simulink library "PTOSim_Lib_Updated"  (R2020b)
settings: Solver=ode45  StartTime=0.0  StopTime=10.0  RelTol=1e-3  EnableMultiTasking=on
undefined symbols (not defined in the file or in its folder): DiscIntNeverNeededParam, pAeq, pAupper_limit, pBeq, pBupper_limit, ptosim, table
libraries: simulink x2, $bdroot x1
(part 1 of 2)
settings Model: RequirementInfo="{}  %GIDa_42666abb_d6d9_408c_ae24_f6520282b61c"  Creator=sor  LastModifiedBy=jleonqu
settings DataIOCC: LimitDataPoints=on  SaveFormat=Array  ReturnWorkspaceOutputs=off
settings OptimizationCC: LifeSpan=inf
settings DebuggingCC: SolverPrmCheckMsg=warning  AllowSymbolicDim=off  SFUnexpectedBacktrackingDiag=warning  SFNoUnconditionalDefaultTransitionDiag=warning  SFExecutionAtInitializationDiag=none  ArithmeticOperatorsInVariantConditions=warning
settings HardwareCC: ProdBitPerPointer=32  ProdBitPerSizeT=32  ProdBitPerPtrDiffT=32  ProdLargestAtomicFloat=None  ProdIntDivRoundTo=Undefined  ProdEndianess=Unspecified  ProdWordSize=32  ProdHWDeviceType=32-bit Generic
settings ModelReferenceCC: PropagateSignalLabelsOutOfModel=off
settings SFSimCC: SimUseLocalCustomCode=off  CustomCodeUndefinedFunction=UseInterfaceOnly
settings RTWCC: RTWUseLocalCustomCode=off
settings CodeAppCC: StateflowObjectComments=on
settings GRTTargetCC: TargetLangStandard=C89/C90 (ANSI)
settings ConfigComp: CovMetricSettings=dw  CovSaveCumulativeToWorkspaceVar=on  CovSaveSingleToWorkspaceVar=on  CovExternalEMLEnable=off  CovSFcnEnable=off

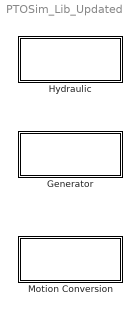
== system PTOSim_Lib_Updated ==
  Generator : Subsystem  RequirementInfo="{}  %GIDa_5439fdb4_7c29_433c_8677_23bf92e18f11"
  Hydraulic : Subsystem  RequirementInfo={} %GIDa_f12a42eb_b9cb_4818_b573_b7dee4183a3b
  Motion Conversion : Subsystem

== system PTOSim_Lib_Updated/Generator ==
  Direct Drive Linear Generator : Subsystem  mask{ptosim=ptosim.pmLinearGenerator(1)}
      mask prompts: ptosim "Machine Name:"
      mask init:
      | if exist ('ptosim','var')
      |     h = [gcb '/To Workspace'];
      |     responseName = ['pmLinearGenerator' num2str(ptosim.number) '_out'];
      |     set_param(h,'VariableName',responseName);
      |     if ischar(ptosim.Rs)==1 ...
      |        || ischar(ptosim.Bfric)==1 ...
      |        || ischar(ptosim.tau_p)==1 ...
      |        || ischar(ptosim.lambda_fd)==1 ...
      |        || ischar(ptosim.Ls)==1 ...
      |        || ischar(ptosim.theta_d_0)==1 ...
      |        || ischar(ptosim.lambda_sq_0)==1 ...
      |        || ischar(ptosim.lambda_sd_0)==1 ...
      |        || ischar(ptosim.Rload) ==1
      |           error('One of the linear generator variables is undefined. For example, ptosim.pmLinearGenerator.variableName')
      |     end       
      | end
      | clear h responseName
  Direct Drive Rotary Generator : Subsystem  RequirementInfo="{}  %GIDa_f3580181_3e4e_42ef_9271_bab532422270"  mask{ptosim=ptosim.pmRotaryGenerator(1)}
      mask prompts: ptosim "Machine Name:"
      mask init:
      | if exist ('ptosim','var')
      |     h = [gcb '/To Workspace'];
      |     responseName = ['pmRotaryGenerator' num2str(ptosim.number) '_out'];
      |     set_param(h,'VariableName',responseName);
      |     if ischar(ptosim.Rs)==1 ...
      |        || ischar(ptosim.Bfric)==1 ...
      |        || ischar(ptosim.tau_p)==1 ...
      |        || ischar(ptosim.lambda_fd)==1 ...
      |        || ischar(ptosim.Ls)==1 ...
      |        || ischar(ptosim.theta_d_0)==1 ...
      |        || ischar(ptosim.lambda_sq_0)==1 ...
      |        || ischar(ptosim.lambda_sd_0)==1 ...
      |        || ischar(ptosim.Rload) ==1 ...
      |        || ischar(ptosim.radius) ==1
      |           error('One of the rotary generator variables is undefined. For example, ptosim.pmRotaryGenerator.variableName')
      |     end       
      | end
      | clear h responseName
  Electric Machine : Subsystem  mask{ptosim=ptosim.ElectricMachine(1), InputFileText=Use PTO-Sim input file to define PTO parameters, Ra=0, La=0, motorConstant=0, ShaftDamping=0, ShaftInertia=0}
      mask prompts: ptosim "Electric Machine Name"; Ra "Armature Resistance [ohm]"; La "Armature Inductance [H]"; motorConstant "Back-emf or Torque constant [V/rpm]"; ShaftDamping "Rotor Damping [N s/m]"; ShaftInertia "Rotor Inertia [kg m^2]"
      settings: PortSchema="{\"entries\":[{\"content\":{\"sides\":[{\"content\":{\"connectorIds\":[\"In1\"]},\"type\":\"ConnectorPlacement.EquallySpacedRectSide\",\"uuid\":\"fc35219d-8831-407a-a01b-8e552e994bd8\"},{\"content\":{\"connectorIds\":[\"Out1\"],\"side\":\"RIGHT\"},\"type\":\"ConnectorPlacement.EquallySpacedRectSide\",\"uuid\":\"8bdf633d-a26b-46f8-9dec-a7b2f777a9d4\"},{\"content\":{\"connectorIds\":[\"In2\"],\"side\":\"TOP\"},\"type\":\"ConnectorPlacement.EquallySpacedRectSide\",\"uuid\":\"317bbc24-ba5c-483d-899e-a231712fee10\"},{\"content\":{\"connectorIds\":[],\"side\":\"HIDDEN\"},\"type\":\"ConnectorPlacement.EquallySpacedRectSide\",\"uuid\":\"59f80c0a-37ef-4cf9-9997-20953bf597e0\"}]},\"type\":\"ConnectorPlacement.EquallySpacedConnector\",\"uuid\":\"aa05d75c-446c-4a7d-9d6c-6346be5c0738\"}],\"packageUris\":[\"http://schema.mathworks.com/mf0/Connector/R2020b\"],\"version\":\"1.0\"}"
      mask DialogControl ParameterGroupVar Prompt: Custom Parameters
      mask DialogControl EMParameters Prompt: Electric Machine Parameters
      mask Display: image('ElectricMotor.png'); % Use "Edit Image" on toolstrip to change.
  Rotary Generator Lookup Table : Subsystem  mask{ptosim=ptosim.rotaryGenerator(1)}
      mask prompts: ptosim "Generator Name"
      mask init:
      | if exist ('ptosim','var')
      |    h = [gcb '/To Workspace'];
      |    responseName = ['rotaryGenerator' num2str(ptosim.number) '_out'];
      |    set_param(h,'VariableName',responseName);
      |    if ischar(ptosim.TgenBase)==1 ...
      |       || ischar(ptosim.omegaBase)==1 ...
      |       || ischar(ptosim.driveEff)==1 ...
      |       || ischar(ptosim.desiredSpeed)==1
      |          error('One of the rotary generator variables is undefined. For example, ptosim.rotaryGenerator.variableName')
      |    end
      | end
      | clear h responseName

== system PTOSim_Lib_Updated/Hydraulic ==
  Accumulator : Subsystem  mask(PTO-Sim Element){ptosim=ptosim.accumulator(1)}
      mask prompts: ptosim "Accumulator Name:"
      mask init:
      | if exist('ptosim','var')
      |     h = [gcb '/To Workspace'];
      |     responseName = ['accumulator' num2str(ptosim.number) '_out'];
      |     set_param(h,'VariableName',responseName);
      |     if ischar(ptosim.VI0)==1 ...
      |             || ischar(ptosim.pIrated)==1 ...
      |             || ischar(ptosim.pIupper_limit)==1 ...
      |             || ischar(ptosim.pIlower_limit)==1 ...
      |             || ischar(ptosim.pIprecharge)==1 ...
      |             || ischar(ptosim.VImax)==1 ...
      |             || ischar(ptosim.VImin)==1 ...
      |             || ischar(ptosim.VIeq)==1 ...
      |             || ischar(ptosim.pIeq)==1 ...
      |             error('One of the accumulator variables is undefined. For example, ptosim.accumulator.variableName')
      |     end
      | end
      | clear h responseName
  Compressible Fluid Piston : Subsystem  mask{ptosim=ptosim.pistonCF(1)}
      mask prompts: ptosim "Piston Name:"
      mask init:
      | if exist ('ptosim','var')
      |     h = [gcb '/To Workspace'];
      |     responseName = ['pistonCF' num2str(ptosim.number) '_out'];
      |     set_param(h,'VariableName',responseName);
      |     
      |     if ischar(ptosim.Ap)==1 ...
      |       || ischar(ptosim.Vo)==1 ...
      |       || ischar(ptosim.Beta_e)==1 ...
      |       || ischar(ptosim.pAi)==1 ...
      |       || ischar(ptosim.pBi)==1 
      |          error('One of the piston variables is undefined. For example, ptosim.pistonCF.variableName')    
      |     end
      | end
      | clear h responseName
  Compressible Fluid Piston Updated : Subsystem  mask{ptosim=ptosim.pistonCF(1), InputFileText=Use PTO-Sim input file to define PTO parameters, Ap_A=0, Ap_B=0, PistonStroke=0, BulkModulus=0, xi_piston=0, pAi=0, pBi=0}
      mask prompts: ptosim "Piston Name"; Ap_A "Piston area A [m]"; Ap_B "Piston area V [m]"; PistonStroke "Piston stroke [m]"; BulkModulus "Fluid Bulk Modulus [Pa]"; xi_piston "Piston initial displacement from A [m]"; pAi "Port A Initial pressure [Pa]"; pBi "Port B Initial pressure [Pa]"
      mask help:
      | PTO-Sim Compressible Fluid Piston
      |
      | This block simualtes a hydraulic cylinder using a compressible fluid model. The block inputs are Response and HydraulicInput. Response is the signal output of the block Rotational PTO Actuation Force. HydraulicInput is a two signal vector with the information of the flow rate for port A and port B of the cylinder. The output of the block is PistonOutput, which is a three signal vector with PressureA, PressureB, and ForcePTO.
      mask init: same as PTOSim_Lib_Updated/Hydraulic/Compressible Fluid Piston
      settings: PortSchema="{\"entries\":[{\"content\":{\"sides\":[{\"content\":{\"connectorIds\":[\"In1\"]},\"type\":\"ConnectorPlacement.EquallySpacedRectSide\",\"uuid\":\"c8df0997-125e-484b-91e1-8ba4eadd9153\"},{\"content\":{\"connectorIds\":[\"Out1\"],\"side\":\"RIGHT\"},\"type\":\"ConnectorPlacement.EquallySpacedRectSide\",\"uuid\":\"941eb644-8b58-45e1-b334-77edb1550c04\"},{\"content\":{\"connectorIds\":[\"In2\"],\"side\":\"TOP\"},\"type\":\"ConnectorPlacement.EquallySpacedRectSide\",\"uuid\":\"a73e5632-eedc-448d-9008-671742bb1d71\"},{\"content\":{\"connectorIds\":[],\"side\":\"HIDDEN\"},\"type\":\"ConnectorPlacement.EquallySpacedRectSide\",\"uuid\":\"aff918e7-82cf-4cd9-bf12-32a09e9272a3\"}]},\"type\":\"ConnectorPlacement.EquallySpacedConnector\",\"uuid\":\"3f3f511d-44ea-4688-8800-5cd126269ecd\"}],\"packageUris\":[\"http://schema.mathworks.com/mf0/Connector/R2020b\"],\"version\":\"1.0\"}"
      mask Help:
      | This block simualtes a hydraulic cylinder using a compressible fluid model. The block inputs are Response and HydraulicInput. Response is the signal output of the block Rotational PTO Actuation Force. HydraulicInput is a two signal vector with the information of the flow rate for port A and port B of the cylinder. The output of the block is PistonOutput, which is a three signal vector with PressureA, PressureB, and ForcePTO.
      | 
      | The outputs are calculated using the model presented in the following link: http://wec-sim.github.io/WEC-Sim/master/user/advanced_features.html#pto-sim
      mask DialogControl ParameterGroupVar Prompt: Custom Parameters
      mask DialogControl PistonProperties Prompt: Piston Properties
      mask DialogControl InitialConditions Prompt: Initial Conditions
      mask Display: image('DoubleActingPiston.png'); % Use "Edit Image" on toolstrip to change.
  Gas-Charged Hydraulic Accumulator : Subsystem  mask{ptosim=ptosim.accumulator(1), InputFileText=Use PTO-Sim input file to define PTO parameters, VI0=0, VIeq=0, pIprecharge=0}
      mask prompts: ptosim "Accumulator Name"; VI0 "Total Volume [m^3]"; VIeq "Initial Volume [m^3]"; pIprecharge "Precharge [Pa]"
      mask DialogControl ParameterGroupVar Prompt: Custom Parameters
      mask DialogControl AccProperties Prompt: Accumulator Properties
      mask Display: image('GasAccumulator.png'); % Use "Edit Image" on toolstrip to change.
  "Hydraulic Motor " : Subsystem  mask{ptosim=ptosim.hydraulicMotor(1)}
      mask prompts: ptosim "Motor Name:"
      mask init:
      | if exist ('ptosim','var')
      |     h = [gcb '/To Workspace'];
      |     responseName = ['hydraulicMotor' num2str(ptosim.number) '_out'];
      |     set_param(h,'VariableName',responseName);
      |     if ischar(ptosim.angVelInit)==1 ...
      |        || ischar(ptosim.J)==1 ...
      |        || ischar(ptosim.fric)==1 ...
      |           error('One of the motor variables is undefined. For example, ptosim.hydraulicMotor.variableName')
      |     end       
      | end
      | clear h responseName
  Noncompressible Fluid Piston : Subsystem  mask{ptosim=ptosim.pistonNCF(1)}
      mask prompts: ptosim "Piston Name:"
      mask init:
      | if exist ('ptosim','var')
      |     h = [gcb '/To Workspace'];
      |     responseName = ['pistonNCF' num2str(ptosim.number) '_out'];
      |     set_param(h,'VariableName',responseName);
      |     if ischar(ptosim.topA)==1 ...
      |       || ischar(ptosim.botA)==1
      |          error('One of the piston variables is undefined. For example, ptosim.pistonNCF.variableName')
      |     end
      | end
      | clear h responseName
  Rectifying Check Valve : Subsystem  mask{ptosim=ptosim.checkValve(1)}
      mask prompts: ptosim "Valve Name:"
      mask init:
      | if exist ('ptosim','var')
      |     h = [gcb '/To Workspace'];
      |     responseName = ['checkValve' num2str(ptosim.number) '_out'];
      |     set_param(h,'VariableName',responseName);
      |     
      |     if ischar(ptosim.Cd)==1 ...
      |        || ischar(ptosim.Amax)==1 ...
      |        || ischar(ptosim.Amin)==1 ...
      |        || ischar(ptosim.pMax)==1 ...
      |        || ischar(ptosim.pMin)==1 ...
      |        || ischar(ptosim.rho)==1 ...
      |        || ischar(ptosim.k1)==1 ...
      |        || ischar(ptosim.k2)==1 
      |           error('One of valve variables is undefined. For exmaple, ptosim.checkValve.variableName')
      |     end
      | end
      | clear h responseName
  Rectifying Valve : Subsystem  mask{ptosim=ptosim.valve(1)}
      mask prompts: ptosim "Valve Name:"
      mask init:
      | if exist ('ptosim','var')
      |     h = [gcb '/To Workspace'];
      |     responseName = ['valve' num2str(ptosim.number) '_out'];
      |     set_param(h,'VariableName',responseName);
      | end
      | clear h responseName

== system PTOSim_Lib_Updated/Motion Conversion ==
  Rotary to Linear Adjustable Rod : Subsystem  mask{ptosim=ptosim.motionMechanism(1)}
      mask prompts: ptosim "Telescope Name:"
      mask init:
      | if exist('ptosim','var')
      |     h = [gcb '/To Workspace'];
      |     responseName = ['motionMechanism' num2str(ptosim.number) '_out'];
      |     set_param(h,'VariableName',responseName);
      |     if ischar(ptosim.crank)==1 ...
      |             || ischar(ptosim.rodInit)==1 ...
      |             || ischar(ptosim.offset)==1 ...
      |             error('One of the rotary to linear adjustable rod variables is undefined. For example, ptosim.motionMechanism.variableName')
      |     end
      | end
      | clear h responseName
  Rotary to Linear Crank : Subsystem  mask{ptosim=ptosim.motionMechanism(1)}
      mask prompts: ptosim "Crank Name:"
      mask init:
      | if exist('ptosim','var')
      |     h = [gcb '/To Workspace'];
      |     responseName = ['motionMechanism' num2str(ptosim.number) '_out'];
      |     set_param(h,'VariableName',responseName);
      |     if ischar(ptosim.crank)==1 ...
      |             || ischar(ptosim.rodLength)==1 ...
      |             || ischar(ptosim.offset)==1 ...
      |             error('One of the rotary to linear crank variables is undefined. For example, ptosim.motionMechanism.variableName')
      |     end
      | end
      | clear h responseName

== system PTOSim_Lib_Updated/Generator/Direct Drive Linear Generator ==
  note: In this model d-axis aligned with rotor magnets
      | in other words lambda_fq = 0
  note: Ls = 3/2*Lsinglephase
  vel : Inport
  ABC2DQ1 : Subsystem
  ABC2DQ2 : Subsystem
  Bus Creator : BusCreator  Inputs=11
  Demux : Demux  Outputs=3
  Demux1 : Demux  Outputs=3
  Gain4 : Gain  Gain=-1
  Gain5 : Gain  Gain=2*pi/(2*ptosim.tau_p)
  Integrator2 : Integrator  InitialCondition=ptosim.theta_d_0
  Load : Subsystem
  Losses : Subsystem
  Product1 : Product
  Subsystem : Subsystem
  Sum : Sum
  Terminator3 : Terminator
  To Workspace : ToWorkspace  VariableName=pmLinearGenerator1_out  SaveFormat=Structure With Time  SampleTime=-1
      settings: Decimation=round(simu.dtOut/simu.dt,0)
  force : Outport
  wires:
  ABC2DQ2/1(DQ) -> Subsystem/1(vsdq)  "vsdq"
  ABC2DQ1/1(abc) -> Demux/1, Load/1(Iabc)  "Iabc"
  Gain5/1 -> Subsystem/2(wd), Integrator2/1  "wsyn"
  Integrator2/1 -> ABC2DQ2/1(theta_d), ABC2DQ1/1(theta_d)
  Product1/1 -> Gain4/1
  Gain4/1 -> Bus Creator/1, Terminator3/1  "absPower"
  Subsystem/1(Fem) -> Sum/2
  Subsystem/2(isdq) -> ABC2DQ1/2(dq)
  Losses/1(friceForce) -> Bus Creator/3, Sum/1  "fricForce"
  Sum/1 -> Bus Creator/2, Product1/2, force/1  "force"
  Load/1(Vabc) -> Demux1/1, ABC2DQ2/2(ABC)  "Vabc"
  vel/1 -> Bus Creator/10, Losses/1(vel), Product1/1, Gain5/1  "vel"
  Bus Creator/1 -> To Workspace/1
  Demux/1 -> Bus Creator/4  "Ia"
  Demux/2 -> Bus Creator/5  "Ib"
  Demux/3 -> Bus Creator/6  "Ic"
  Demux1/1 -> Bus Creator/7  "Va"
  Demux1/2 -> Bus Creator/8  "Vb"
  Demux1/3 -> Bus Creator/9  "Vc"
  Load/2(elecPower) -> Bus Creator/11  "elecPower"

== system PTOSim_Lib_Updated/Generator/Direct Drive Rotary Generator ==
  note: In this model d-axis aligned with rotor magnets
      | in other words lambda_fq = 0
  note: Ls = 3/2*Lsinglephase
  vel : Inport
  ABC2DQ1 : Subsystem
  ABC2DQ2 : Subsystem
  Bus Creator : BusCreator  Inputs=11
  Demux : Demux  Outputs=3
  Demux1 : Demux  Outputs=3
  Gain4 : Gain  Gain=-1
  Gain5 : Gain  Gain=2*pi*ptosim.radius/(2*ptosim.tau_p)
  Integrator2 : Integrator  InitialCondition=ptosim.theta_d_0
  Load : Subsystem
  Losses : Subsystem
  Product1 : Product
  Subsystem : Subsystem
  Sum : Sum
  Terminator3 : Terminator
  To Workspace : ToWorkspace  VariableName=pmRotaryGenerator1_out  SaveFormat=Structure With Time  SampleTime=-1
      settings: Decimation=round(simu.dtOut/simu.dt,0)
  torque : Outport
  wires:
  ABC2DQ2/1(DQ) -> Subsystem/1(vsdq)  "vsdq"
  ABC2DQ1/1(abc) -> Demux/1, Load/1(Iabc)  "Iabc"
  Gain5/1 -> Integrator2/1, Subsystem/2(wd)  "wsyn"
  Integrator2/1 -> ABC2DQ2/1(theta_d), ABC2DQ1/1(theta_d)
  Product1/1 -> Gain4/1
  Gain4/1 -> Bus Creator/1, Terminator3/1  "absPower"
  Subsystem/1(Tem) -> Sum/2
  Subsystem/2(isdq) -> ABC2DQ1/2(dq)
  Losses/1(fricTorque) -> Bus Creator/3, Sum/1  "fricTorque"
  Sum/1 -> Bus Creator/2, Product1/2, torque/1  "torque"
  Load/1(Vabc) -> Demux1/1, ABC2DQ2/2(ABC)  "Vabc"
  vel/1 -> Losses/1(vel), Product1/1, Gain5/1, Bus Creator/10  "vel"
  Bus Creator/1 -> To Workspace/1
  Demux/1 -> Bus Creator/4  "Ia"
  Demux/2 -> Bus Creator/5  "Ib"
  Demux/3 -> Bus Creator/6  "Ic"
  Demux1/1 -> Bus Creator/7  "Va"
  Demux1/2 -> Bus Creator/8  "Vb"
  Demux1/3 -> Bus Creator/9  "Vc"
  Load/2(elecPower) -> Bus Creator/11  "elecPower"

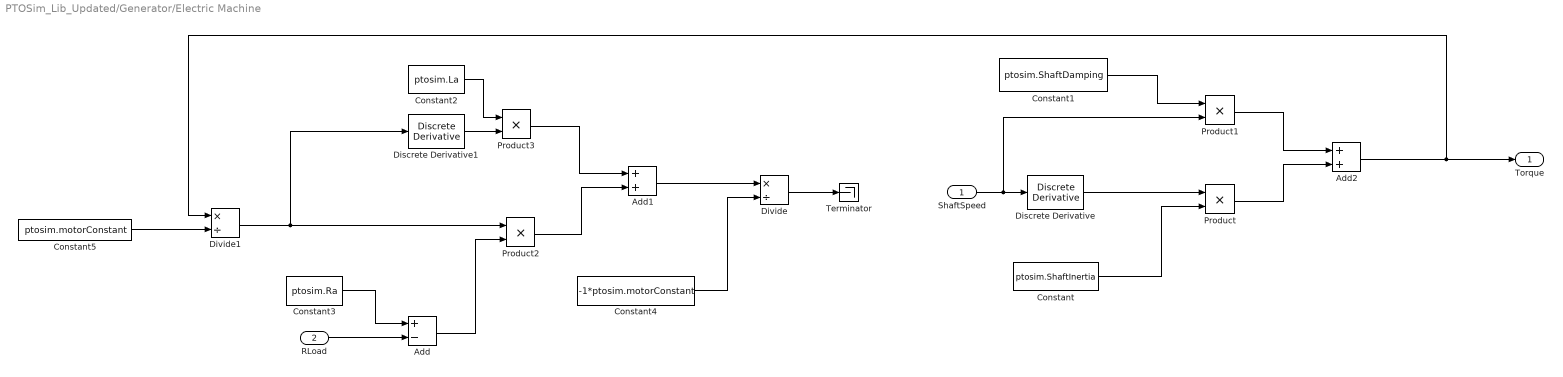
== system PTOSim_Lib_Updated/Generator/Electric Machine ==
  ShaftSpeed : Inport
  RLoad : Inport  Port=2
  Add : Sum  Inputs=+-
  Add1 : Sum
  Add2 : Sum
  Constant : Constant  Value=ptosim.ShaftInertia
  Constant1 : Constant  Value=ptosim.ShaftDamping
  Constant2 : Constant  Value=ptosim.La
  Constant3 : Constant  Value=ptosim.Ra
  Constant4 : Constant  Value=-1*ptosim.motorConstant
  Constant5 : Constant  Value=ptosim.motorConstant
  Discrete Derivative : simulink/Discrete/Discrete Derivative  gainval=1.0  ICPrevScaledInput=0.0  OutMin=[]  OutMax=[]  OutDataType=fixdt(1, 16)  OutScaling=2^-10  DoSatur=off
  Discrete Derivative1 : simulink/Quick Insert/Discrete/Discrete Derivative  gainval=1.0  ICPrevScaledInput=0.0  OutMin=[]  OutMax=[]  OutDataType=fixdt(1, 16)  OutScaling=2^-10  DoSatur=off
      settings: SourceProductBaseCode=SL
  Divide : Product  Inputs=*/
  Divide1 : Product  Inputs=*/
  Product{,1..3} (4 alike) : Product
  Terminator : Terminator
  Torque : Outport
  wires:
  Discrete Derivative/1 -> Product/1
  Constant/1 -> Product/2
  Constant1/1 -> Product1/1
  Divide1/1 -> Discrete Derivative1/1, Product2/1
  RLoad/1 -> Add/2
  Constant3/1 -> Add/1
  Add/1 -> Product2/2
  Discrete Derivative1/1 -> Product3/2
  Constant2/1 -> Product3/1
  Product3/1 -> Add1/1
  Product2/1 -> Add1/2
  Add1/1 -> Divide/1
  Constant4/1 -> Divide/2
  Product1/1 -> Add2/1
  Product/1 -> Add2/2
  Add2/1 -> Divide1/1, Torque/1
  ShaftSpeed/1 -> Product1/2, Discrete Derivative/1
  Constant5/1 -> Divide1/2
  Divide/1 -> Terminator/1

== system PTOSim_Lib_Updated/Generator/Rotary Generator Lookup Table ==
  delPress : Inport
  motorVol : Inport  Port=2
  angVel : Inport  Port=3
  Base Motor Torque : Gain  Gain=-1/ptosim.TgenBase
  Base Motor Torque1 : Gain  Gain=1/ptosim.omegaBase
  Base Motor Torque2 : Gain  Gain=ptosim.driveEff
  Base Motor Torque3 : Gain  Gain=1/100
  Base Motor Torque4 : Gain  Gain=1.05
  Bus Creator : BusCreator  Inputs=2
  Constant47 : Constant  Value=ptosim.desiredSpeed
  Divide1 : Product  Inputs=*/
  PM p.u. Efficiency Lookup Table : Lookup_n-D  BreakpointsForDimension1=table.Tpu(:,1)  BreakpointsForDimension2=table.omegapu(1,:)  Table=table.eff  InterpMethod=Flat  InputSameDT=on
      settings: InputPortMap=u0,u1
  Product{,1..3} (4 alike) : Product  RndMeth=Zero
  To Workspace : ToWorkspace  VariableName=rotaryGenerator1_out  SaveFormat=Structure With Time  SampleTime=-1
      settings: Decimation=round(simu.dtOut/simu.dt,0)
  genTorque : Outport
  wires:
  angVel/1 -> Product2/2, Product/2, Base Motor Torque1/1
  Product2/1 -> Product/1, Base Motor Torque/1, genTorque/1
  Bus Creator/1 -> To Workspace/1
  Base Motor Torque/1 -> PM p.u. Efficiency Lookup Table/1  "torquePU"
  Base Motor Torque1/1 -> PM p.u. Efficiency Lookup Table/2  "omegaPU"
  PM p.u. Efficiency Lookup Table/1 -> Base Motor Torque3/1
  Base Motor Torque3/1 -> Product1/2  "genEff"
  Product/1 -> Product1/1, Bus Creator/2  "genPower"
  Product1/1 -> Base Motor Torque2/1
  Base Motor Torque2/1 -> Bus Creator/1  "elecPower"
  Divide1/1 -> Product2/1
  delPress/1 -> Product3/1
  motorVol/1 -> Product3/2
  Product3/1 -> Divide1/1
  Constant47/1 -> Base Motor Torque4/1
  Base Motor Torque4/1 -> Divide1/2

== system PTOSim_Lib_Updated/Hydraulic/Accumulator ==
  volFlowM : Inport
  volFlowAccum : Inport  Port=2
  Bus Creator : BusCreator  Inputs=2
  Constant : Constant
  Constant3 : Constant  Value=ptosim.pIprecharge
  Constant4 : Constant  Value=ptosim.VI0
  Divide : Product  Inputs=*/
  Divide1 : Product  Inputs=*/
  Exponent : Constant  Value=1.4
  Integrator4 : Integrator  InitialCondition=ptosim.VIeq
  Math Function : Math  Operator=pow  SignedPower=on  SaturateOnIntegerOverflow=on
  Sum : Sum  Inputs=-+
  Sum2 : Sum
  To Workspace : ToWorkspace  VariableName=accum_out  SaveFormat=Structure With Time  SampleTime=-1
      settings: Decimation=round(simu.dtOut/simu.dt,0)
  pressure : Outport
  wires:
  Sum2/1 -> Integrator4/1
  Integrator4/1 -> Bus Creator/2, Divide/1  "volume"
  Constant4/1 -> Divide/2
  Constant/1 -> Sum/2
  Divide/1 -> Sum/1
  Exponent/1 -> Math Function/2
  Sum/1 -> Math Function/1
  Math Function/1 -> Divide1/2
  Constant3/1 -> Divide1/1
  Divide1/1 -> pressure/1, Bus Creator/1  "pressure"
  volFlowAccum/1 -> Sum2/2
  volFlowM/1 -> Sum2/1
  Bus Creator/1 -> To Workspace/1

== system PTOSim_Lib_Updated/Hydraulic/Compressible Fluid Piston ==
  pos : Inport
  vel : Inport  Port=2
  volFlowTop : Inport  Port=3
  volFlowBottom : Inport  Port=4
  Bus Creator : BusCreator  Inputs=4
  Gain1 : Gain  Gain=-1
  Gain6 : Gain  Gain=ptosim.Ap
  Gain7 : Gain  Gain=ptosim.Ap
  Pressure Bottom : Subsystem
  Pressure Top : Subsystem
  Product : Product
  Sum4 : Sum  Inputs=-+
  To Workspace : ToWorkspace  VariableName=pistonCF1_out  SaveFormat=Structure With Time  SampleTime=-1
      settings: Decimation=round(simu.dtOut/simu.dt,0)
  force : Outport
  topPressure : Outport  Port=2
  bottomPressure : Outport  Port=3
  wires:
  Pressure Top/1(topPressure) -> Sum4/1, topPressure/1
  Pressure Bottom/1(bottomPressure) -> bottomPressure/1, Sum4/2
  Gain7/1 -> Pressure Bottom/3(volFLowP), Pressure Top/3(volFlowP)
  pos/1 -> Bus Creator/3, Pressure Bottom/1(pos), Pressure Top/1(pos)  "pos"
  vel/1 -> Bus Creator/4, Product/2, Gain7/1  "vel"
  Sum4/1 -> Gain6/1
  Gain6/1 -> Bus Creator/2, force/1, Product/1  "force"
  volFlowBottom/1 -> Pressure Bottom/2(volFlowBottom)
  volFlowTop/1 -> Pressure Top/2(volFlowTop)
  Bus Creator/1 -> To Workspace/1
  Gain1/1 -> Bus Creator/1  "absPower"
  Product/1 -> Gain1/1

== system PTOSim_Lib_Updated/Hydraulic/Compressible Fluid Piston Updated ==
  HydraulicInput : Inport
  Response : Inport  Port=2
  Add : Sum  Inputs=-+
  Bus Creator : BusCreator  Inputs=3
  Bus Selector : BusSelector  OutputSignals=position,velocity
  Bus Selector1 : BusSelector  OutputSignals=QA,QB
  Constant : Constant  Value=ptosim.Ap_B
  Constant1 : Constant  Value=ptosim.Ap_A
  Discrete-Time Integrator : DiscreteIntegrator  InitialCondition=ptosim.pAi  SampleTime=-1  ICPrevOutput=DiscIntNeverNeededParam  ICPrevScaledInput=DiscIntNeverNeededParam
  Discrete-Time Integrator1 : DiscreteIntegrator  InitialCondition=ptosim.pBi  SampleTime=-1  ICPrevOutput=DiscIntNeverNeededParam  ICPrevScaledInput=DiscIntNeverNeededParam
  Product1 : Product
  Product2 : Product
  Selector : Selector  InputPortWidth=6  IndexOptions=Index vector (dialog)  Indices=3  OutputSizes=1
  Selector1 : Selector  InputPortWidth=6  IndexOptions=Index vector (dialog)  Indices=3  OutputSizes=1
  Subsystem : Subsystem  AncestorBlock=PTOSim_Lib_Updated/Hydraulic/Compressible Fluid Piston Updated/Subsystem
  dPa_dt : Subsystem  AncestorBlock=PTOSim_Lib_Updated/Hydraulic/Compressible Fluid Piston Updated/dPa_dt
  PistonOutput : Outport
  wires:
  Bus Selector/1 -> Selector/1  "<position>"
  Product1/1 -> Add/2
  HydraulicInput/1 -> Bus Selector1/1
  Subsystem/1(dPB_dt) -> Discrete-Time Integrator1/1
  dPa_dt/1(dPA_dt) -> Discrete-Time Integrator/1
  Product2/1 -> Add/1
  Selector/1 -> Subsystem/1(Pos), dPa_dt/1(Pos)
  Discrete-Time Integrator/1 -> Bus Creator/1, Product2/1  "PressureA"
  Response/1 -> Bus Selector/1
  Selector1/1 -> Subsystem/2(Vel), dPa_dt/2(Vel)
  Discrete-Time Integrator1/1 -> Bus Creator/3, Product1/2  "ForcePTO"
  Bus Selector/2 -> Selector1/1  "<velocity>"
  Constant/1 -> Product1/1
  Constant1/1 -> Product2/2
  Add/1 -> Bus Creator/2  "PressureB"
  Bus Creator/1 -> PistonOutput/1
  Bus Selector1/2 -> Subsystem/3(QB)  "<QB>"
  Bus Selector1/1 -> dPa_dt/3(QA)  "<QA>"

== system PTOSim_Lib_Updated/Hydraulic/Gas-Charged Hydraulic Accumulator ==
  FlowRate : Inport
  Add : Sum  Inputs=+-
  Constant : Constant  Value=ptosim.VI0
  Constant1 : Constant
  Constant2 : Constant  Value=1.4
  Constant3 : Constant  Value=ptosim.pIprecharge
  Discrete-Time Integrator : DiscreteIntegrator  InitialCondition=ptosim.VIeq  SampleTime=-1  ICPrevOutput=DiscIntNeverNeededParam  ICPrevScaledInput=DiscIntNeverNeededParam
  Divide : Product  Inputs=*/
  Divide1 : Product  Inputs=*/
  Math Function : Math  Operator=pow  SaturateOnIntegerOverflow=on
  Pressure : Outport
  wires:
  FlowRate/1 -> Discrete-Time Integrator/1
  Discrete-Time Integrator/1 -> Divide/1
  Constant/1 -> Divide/2
  Divide/1 -> Add/2
  Constant1/1 -> Add/1
  Add/1 -> Math Function/1
  Constant2/1 -> Math Function/2
  Math Function/1 -> Divide1/2
  Constant3/1 -> Divide1/1
  Divide1/1 -> Pressure/1

== system PTOSim_Lib_Updated/Hydraulic/Hydraulic Motor  ==
  highPressure : Inport
  lowPressure : Inport  Port=2
  genTorque : Inport  Port=3
  Bus Creator : BusCreator  Inputs=2
  Constant47 : Constant  Value=ptosim.J
  Divide1 : Product  Inputs=*/
  Gain1 : Gain  Gain=ptosim.fric
  Gain4 : Gain  Gain=-1
  Integrator1 : Integrator  InitialCondition=ptosim.angVelInit
  Interpreted MATLAB Function : MATLABFcn  MATLABFcn=variableMotorVolume
  Product : Product
  Product1 : Product
  Sum1 : Sum  Inputs=+--
  Sum2 : Sum  Inputs=+-
  To Workspace : ToWorkspace  VariableName=hydraulicMotor1_out  SaveFormat=Structure With Time  SampleTime=-1
      settings: Decimation=round(simu.dtOut/simu.dt,0)
  delPress : Outport
  motorVol : Outport  Port=2
  angVel : Outport  Port=3
  volFlowMHigh : Outport  Port=4
  volFlowMLow : Outport  Port=5
  wires:
  Interpreted MATLAB Function/1 -> motorVol/1, Product/2, Product1/2
  Sum2/1 -> delPress/1, Product/1, Interpreted MATLAB Function/1
  Gain1/1 -> Sum1/3
  genTorque/1 -> Sum1/2, Gain1/1
  Bus Creator/1 -> To Workspace/1
  Gain4/1 -> volFlowMHigh/1
  lowPressure/1 -> Sum2/2
  highPressure/1 -> Sum2/1
  Integrator1/1 -> angVel/1, Product1/1, Bus Creator/1  "angVel"
  Divide1/1 -> Integrator1/1
  Constant47/1 -> Divide1/2
  Sum1/1 -> Divide1/1
  Product/1 -> Sum1/1
  Product1/1 -> volFlowMLow/1, Gain4/1, Bus Creator/2  "volFlowM"

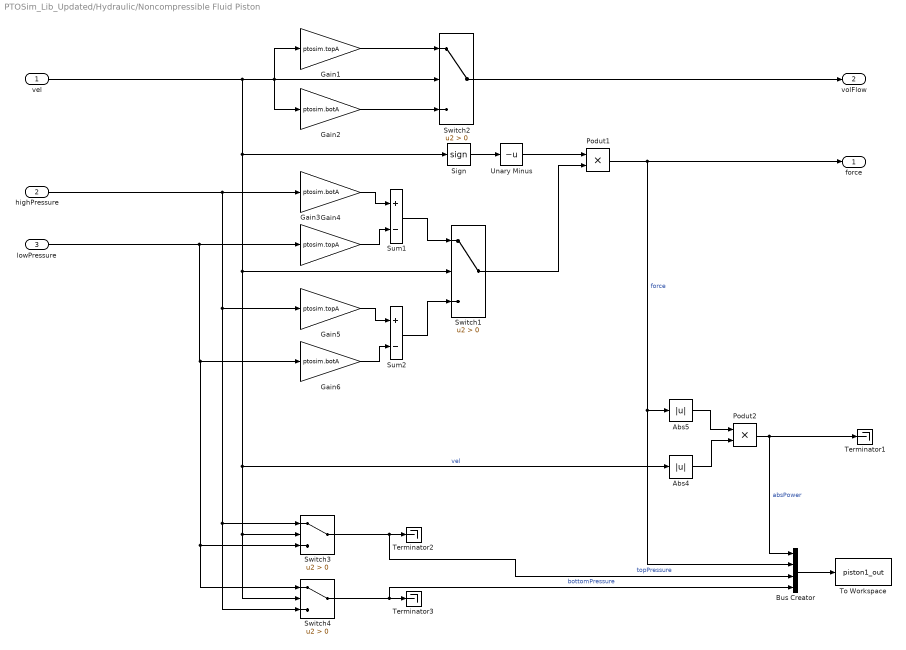
== system PTOSim_Lib_Updated/Hydraulic/Noncompressible Fluid Piston ==
  vel : Inport
  highPressure : Inport  Port=2
  lowPressure : Inport  Port=3
  Abs4 : Abs
  Abs5 : Abs
  Bus Creator : BusCreator  Inputs=4
  Gain1 : Gain  Gain=ptosim.topA
  Gain2 : Gain  Gain=ptosim.botA
  Gain3 : Gain  Gain=ptosim.topA
  Gain4 : Gain  Gain=ptosim.botA
  Gain5 : Gain  Gain=ptosim.topA
  Gain6 : Gain  Gain=ptosim.botA
  Podut1 : Product  RndMeth=Zero
  Podut2 : Product  RndMeth=Zero
  Sign : Signum
  Sum1 : Sum  Inputs=+-
  Sum2 : Sum  Inputs=+-
  Switch{1..4} (4 alike) : Switch  Criteria=u2 > Threshold
  Terminator1 : Terminator
  Terminator2 : Terminator
  Terminator3 : Terminator
  To Workspace : ToWorkspace  VariableName=piston1_out  SaveFormat=Structure With Time  SampleTime=-1
      settings: Decimation=round(simu.dtOut/simu.dt,0)
  Unary Minus : UnaryMinus
  force : Outport
  volFlow : Outport  Port=2
  wires:
  vel/1 -> Switch1/2, Switch4/2, Switch3/2, Abs4/1, Sign/1, Gain2/1, Switch2/2, Gain1/1  "vel"
  Podut2/1 -> Bus Creator/1, Terminator1/1  "absPower"
  Abs5/1 -> Podut2/1
  Abs4/1 -> Podut2/2
  Gain1/1 -> Switch2/1
  Gain2/1 -> Switch2/3
  Sum1/1 -> Switch1/1
  Podut1/1 -> force/1, Bus Creator/2, Abs5/1  "force"
  Gain4/1 -> Sum1/1
  Gain3/1 -> Sum1/2
  highPressure/1 -> Gain5/1, Switch3/1, Switch4/3, Gain4/1
  lowPressure/1 -> Switch4/1, Switch3/3, Gain6/1, Gain3/1
  Gain5/1 -> Sum2/1
  Gain6/1 -> Sum2/2
  Sum2/1 -> Switch1/3
  Sign/1 -> Unary Minus/1
  Unary Minus/1 -> Podut1/1
  Switch1/1 -> Podut1/2
  Switch3/1 -> Bus Creator/3, Terminator2/1  "topPressure"
  Switch4/1 -> Bus Creator/4, Terminator3/1  "bottomPressure"
  Switch2/1 -> volFlow/1
  Bus Creator/1 -> To Workspace/1

== system PTOSim_Lib_Updated/Hydraulic/Rectifying Check Valve ==
  topPressure : Inport
  bottomPressure : Inport  Port=2
  highPressure : Inport  Port=3
  lowPressure : Inport  Port=4
  Bus Creator : BusCreator  Inputs=4
  Subsystem : Subsystem
  Subsystem1 : Subsystem
  Subsystem2 : Subsystem
  Subsystem3 : Subsystem
  Sum1 : Sum  Inputs=-+
  Sum2 : Sum
  Sum3 : Sum  Inputs=--
  Sum4 : Sum  Inputs=-+
  To Workspace : ToWorkspace  VariableName=valve1_out  SaveFormat=Structure With Time  SampleTime=-1
      settings: Decimation=round(simu.dtOut/simu.dt,0)
  volFlowTop : Outport
  volFlowBottom : Outport  Port=2
  volFlowHigh : Outport  Port=3
  volFlowLow : Outport  Port=4
  wires:
  topPressure/1 -> Subsystem3/2(topPressure), Subsystem/1(topPressure)
  bottomPressure/1 -> Subsystem2/2(bottomPressure), Subsystem1/1(bottomPressure)
  highPressure/1 -> Subsystem1/2(highPressure), Subsystem/2(highPressure)
  lowPressure/1 -> Subsystem2/1(lowPressure), Subsystem3/1(lowPressure)
  Subsystem3/1(volFlow4) -> Bus Creator/4, Sum4/2, Sum3/2  "volFlow4"
  Subsystem2/1(volFlow3) -> Bus Creator/3, Sum3/1, Sum1/2  "volFlow3"
  Subsystem1/1(volFlow2) -> Bus Creator/2, Sum2/2, Sum1/1  "volFlow2"
  Subsystem/1(volFlow1) -> Bus Creator/1, Sum2/1, Sum4/1  "volFlow1"
  Sum4/1 -> volFlowTop/1
  Sum1/1 -> volFlowBottom/1
  Sum2/1 -> volFlowHigh/1
  Sum3/1 -> volFlowLow/1
  Bus Creator/1 -> To Workspace/1

== system PTOSim_Lib_Updated/Hydraulic/Rectifying Valve ==
  volFlow : Inport
  Abs1 : Abs
  To Workspace : ToWorkspace  VariableName=valve1_out  SaveFormat=Structure With Time  SampleTime=-1
      settings: Decimation=round(simu.dtOut/simu.dt,0)
  electric generator control1 : Gain  Gain=-1
  volFlowHigh : Outport
  volFlowLow : Outport  Port=2
  wires:
  Abs1/1 -> To Workspace/1, volFlowHigh/1, electric generator control1/1  "volFlow"
  electric generator control1/1 -> volFlowLow/1
  volFlow/1 -> Abs1/1

== system PTOSim_Lib_Updated/Motion Conversion/Rotary to Linear Adjustable Rod ==
  angPos : Inport
  angVel : Inport  Port=2
  force : Inport  Port=3
  Add : Sum
  Angle Calculation for PTO : Subsystem
  Angular to Linear Position : Subsystem
  Angular to Linear Velocity : Subsystem
  Bus Creator : BusCreator  Inputs=3
  Constant1 : Constant  Value=ptosim.crank
  Constant2 : Constant  Value=ptosim.crank
  Gain : Gain  Gain=-1
  Product : Product  Inputs=4
  Product1 : Product  Inputs=4
  To Workspace : ToWorkspace  VariableName=motionmech1_out  SaveFormat=Structure With Time  SampleTime=-1
      settings: Decimation=round(simu.dtOut/simu.dt,0)
  Trigonometric Function : Trigonometry
  Trigonometric Function1 : Trigonometry  Operator=cos
  linearPos : Outport
  linearVel : Outport  Port=2
  torque : Outport  Port=3
  wires:
  Angular to Linear Position/1(linearPos) -> linearPos/1
  angVel/1 -> Bus Creator/3, Angular to Linear Velocity/2(angVel)  "angVelocity"
  Angular to Linear Velocity/1(linearVel) -> linearVel/1
  Add/1 -> Bus Creator/1, torque/1  "ptoTorque"
  Bus Creator/1 -> To Workspace/1
  angPos/1 -> Angular to Linear Velocity/1(angPos), Trigonometric Function1/1, Trigonometric Function/1, Angle Calculation for PTO/1(angPos), Bus Creator/2, Angular to Linear Position/1(angPos)  "angPosition"
  Product1/1 -> Add/1
  Gain/1 -> Add/2
  Angle Calculation for PTO/2(Sin_gamma) -> Product/1
  Trigonometric Function1/1 -> Product1/3
  Angle Calculation for PTO/1(Cos_gamma) -> Product1/1
  force/1 -> Product1/4, Product/4
  Constant2/1 -> Product1/2
  Trigonometric Function/1 -> Product/3
  Constant1/1 -> Product/2
  Product/1 -> Gain/1

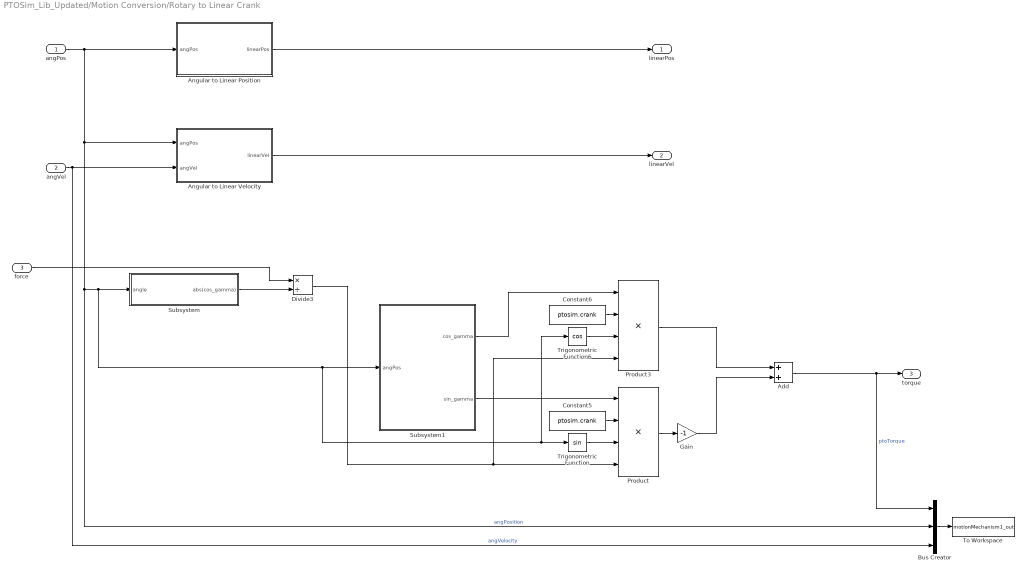
== system PTOSim_Lib_Updated/Motion Conversion/Rotary to Linear Crank ==
  angPos : Inport
  angVel : Inport  Port=2
  force : Inport  Port=3
  Add : Sum
  Angular to Linear Position : Subsystem
  Angular to Linear Velocity : Subsystem
  Bus Creator : BusCreator  Inputs=3
  Constant5 : Constant  Value=ptosim.crank
  Constant6 : Constant  Value=ptosim.crank
  Divide3 : Product  Inputs=*/
  Gain : Gain  Gain=-1
  Product : Product  Inputs=4
  Product3 : Product  Inputs=4
  Subsystem : Subsystem
  Subsystem1 : Subsystem  AncestorBlock=PTOSim_Lib/Motion Conversion/Rotary to Linear Adjustable Rod/Subsystem
  To Workspace : ToWorkspace  VariableName=motionMechanism1_out  SaveFormat=Structure With Time  SampleTime=-1
      settings: Decimation=round(simu.dtOut/simu.dt,0)
  Trigonometric Function : Trigonometry
  Trigonometric Function6 : Trigonometry  Operator=cos
  linearPos : Outport
  linearVel : Outport  Port=2
  torque : Outport  Port=3
  wires:
  Angular to Linear Position/1(linearPos) -> linearPos/1
  angVel/1 -> Bus Creator/3, Angular to Linear Velocity/2(angVel)  "angVelocity"
  Angular to Linear Velocity/1(linearVel) -> linearVel/1
  Add/1 -> Bus Creator/1, torque/1  "ptoTorque"
  Bus Creator/1 -> To Workspace/1
  Subsystem/1(abs(cos_gamma)) -> Divide3/2
  force/1 -> Divide3/1
  Trigonometric Function6/1 -> Product3/3
  Subsystem1/1(cos_gamma) -> Product3/1
  Constant6/1 -> Product3/2
  Divide3/1 -> Product/4, Product3/4
  Gain/1 -> Add/2
  Product3/1 -> Add/1
  Subsystem1/2(sin_gamma) -> Product/1
  angPos/1 -> Angular to Linear Velocity/1(angPos), Subsystem1/1(angPos), Trigonometric Function/1, Trigonometric Function6/1, Subsystem/1(angle), Bus Creator/2, Angular to Linear Position/1(angPos)  "angPosition"
  Trigonometric Function/1 -> Product/3
  Constant5/1 -> Product/2
  Product/1 -> Gain/1

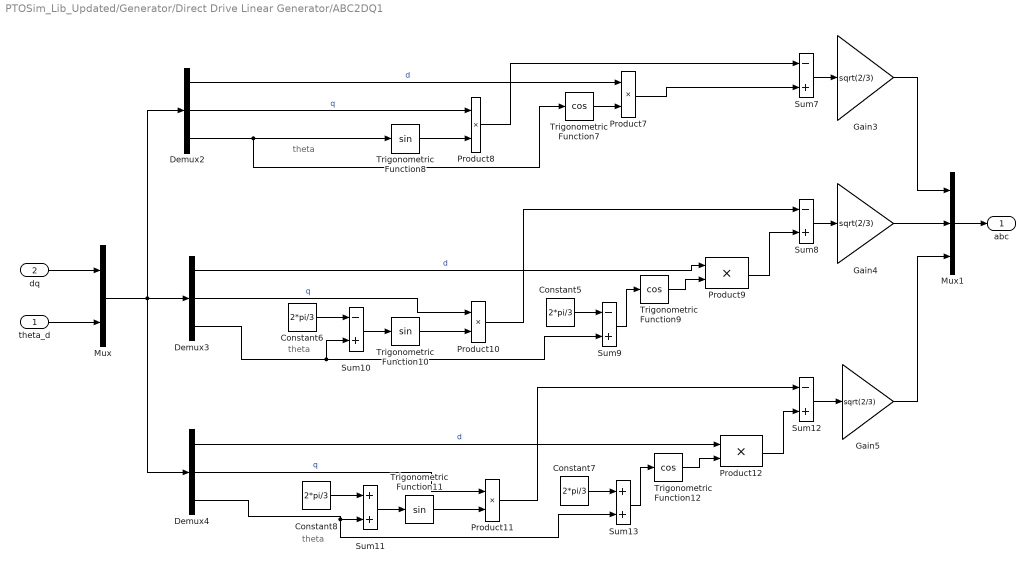
== system PTOSim_Lib_Updated/Generator/Direct Drive Linear Generator/ABC2DQ1 ==
  note: theta
  note: theta
  note: theta
  theta_d : Inport
  dq : Inport  Port=2
  Constant{5..8} (4 alike) : Constant  Value=2*pi/3
  Demux2 : Demux  Outputs=3
      settings: DisplayOption=none
  Demux3 : Demux  Outputs=3
      settings: DisplayOption=none
  Demux4 : Demux  Outputs=3
      settings: DisplayOption=none
  Gain3 : Gain  Gain=sqrt(2/3)  SaturateOnIntegerOverflow=on  OutDataTypeStr=Inherit: Same as input  ParamDataTypeStr=Inherit: Same as input
  Gain4 : Gain  Gain=sqrt(2/3)  SaturateOnIntegerOverflow=on  OutDataTypeStr=Inherit: Same as input  ParamDataTypeStr=Inherit: Same as input
  Gain5 : Gain  Gain=sqrt(2/3)  SaturateOnIntegerOverflow=on  OutDataTypeStr=Inherit: Same as input  ParamDataTypeStr=Inherit: Same as input
  Mux : Mux  Inputs=2
  Mux1 : Mux  Inputs=3
  Product{7..12} (6 alike) : Product  InputSameDT=on  SaturateOnIntegerOverflow=on  OutDataTypeStr=Inherit: Same as first input
  Sum{7..10,12} (5 alike) : Sum  Inputs=-+  InputSameDT=on  SaturateOnIntegerOverflow=on  OutDataTypeStr=Inherit: Same as first input
  Sum11 : Sum  InputSameDT=on  SaturateOnIntegerOverflow=on  OutDataTypeStr=Inherit: Same as first input
  Sum13 : Sum  InputSameDT=on  SaturateOnIntegerOverflow=on  OutDataTypeStr=Inherit: Same as first input
  Trigonometric Function10 : Trigonometry
  Trigonometric Function11 : Trigonometry
  Trigonometric Function12 : Trigonometry  Operator=cos
  Trigonometric Function7 : Trigonometry  Operator=cos
  Trigonometric Function8 : Trigonometry
  Trigonometric Function9 : Trigonometry  Operator=cos
  abc : Outport
  wires:
  Mux1/1 -> abc/1
  dq/1 -> Mux/1
  theta_d/1 -> Mux/2
  Mux/1 -> Demux4/1, Demux2/1, Demux3/1
  Trigonometric Function7/1 -> Product7/2
  Demux2/1 -> Product7/1  "d"
  Product7/1 -> Sum7/2
  Product8/1 -> Sum7/1
  Demux2/3 -> Trigonometric Function8/1, Trigonometric Function7/1
  Demux2/2 -> Product8/1  "q"
  Trigonometric Function9/1 -> Product9/2
  Demux3/1 -> Product9/1  "d"
  Product9/1 -> Sum8/2
  Product10/1 -> Sum8/1
  Demux3/3 -> Sum10/2, Sum9/2
  Trigonometric Function10/1 -> Product10/2
  Demux3/2 -> Product10/1  "q"
  Sum9/1 -> Trigonometric Function9/1
  Constant5/1 -> Sum9/1
  Sum10/1 -> Trigonometric Function10/1
  Constant6/1 -> Sum10/1
  Trigonometric Function12/1 -> Product12/2
  Demux4/1 -> Product12/1  "d"
  Product12/1 -> Sum12/2
  Product11/1 -> Sum12/1
  Demux4/3 -> Sum13/2, Sum11/2
  Trigonometric Function11/1 -> Product11/2
  Demux4/2 -> Product11/1  "q"
  Sum13/1 -> Trigonometric Function12/1
  Constant7/1 -> Sum13/1
  Sum11/1 -> Trigonometric Function11/1
  Constant8/1 -> Sum11/1
  Sum7/1 -> Gain3/1
  Sum8/1 -> Gain4/1
  Sum12/1 -> Gain5/1
  Gain3/1 -> Mux1/1
  Gain4/1 -> Mux1/2
  Gain5/1 -> Mux1/3
  Trigonometric Function8/1 -> Product8/2

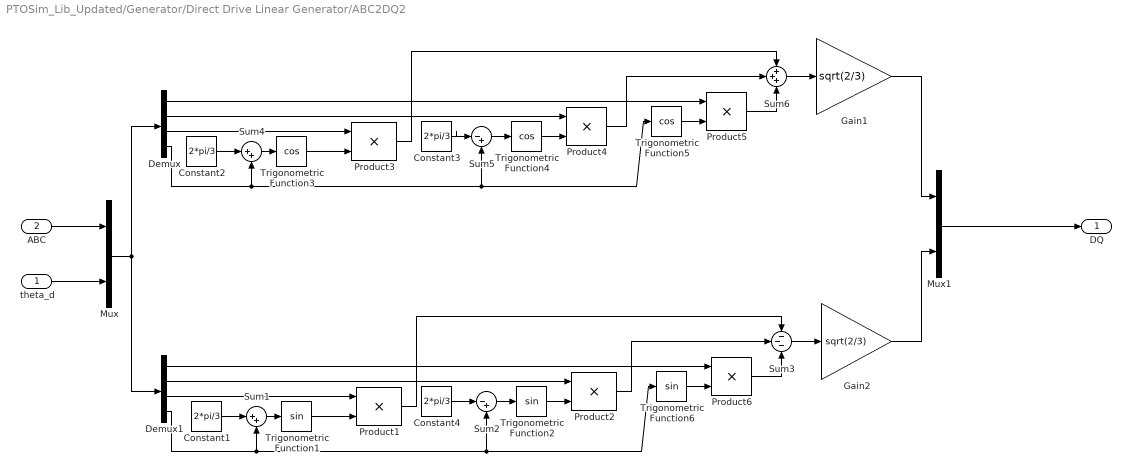
== system PTOSim_Lib_Updated/Generator/Direct Drive Linear Generator/ABC2DQ2 ==
  theta_d : Inport
  ABC : Inport  Port=2
  Constant{1..4} (4 alike) : Constant  Value=2*pi/3
  Demux : Demux
      settings: DisplayOption=none
  Demux1 : Demux
      settings: DisplayOption=none
  Gain1 : Gain  Gain=sqrt(2/3)  SaturateOnIntegerOverflow=on  OutDataTypeStr=Inherit: Same as input  ParamDataTypeStr=Inherit: Same as input
  Gain2 : Gain  Gain=sqrt(2/3)  SaturateOnIntegerOverflow=on  OutDataTypeStr=Inherit: Same as input  ParamDataTypeStr=Inherit: Same as input
  Mux : Mux  Inputs=2
  Mux1 : Mux  Inputs=2
  Product{1..6} (6 alike) : Product  InputSameDT=on  SaturateOnIntegerOverflow=on  OutDataTypeStr=Inherit: Same as first input
  Sum1 : Sum  Inputs=|++  InputSameDT=on  SaturateOnIntegerOverflow=on  OutDataTypeStr=Inherit: Same as first input
  Sum2 : Sum  Inputs=|-+  InputSameDT=on  SaturateOnIntegerOverflow=on  OutDataTypeStr=Inherit: Same as first input
  Sum3 : Sum  Inputs=---  InputSameDT=on  SaturateOnIntegerOverflow=on  OutDataTypeStr=Inherit: Same as first input
  Sum4 : Sum  Inputs=|++  InputSameDT=on  SaturateOnIntegerOverflow=on  OutDataTypeStr=Inherit: Same as first input
  Sum5 : Sum  Inputs=|-+  InputSameDT=on  SaturateOnIntegerOverflow=on  OutDataTypeStr=Inherit: Same as first input
  Sum6 : Sum  Inputs=+++  InputSameDT=on  SaturateOnIntegerOverflow=on  OutDataTypeStr=Inherit: Same as first input
  Trigonometric Function1 : Trigonometry
  Trigonometric Function2 : Trigonometry
  Trigonometric Function3 : Trigonometry  Operator=cos
  Trigonometric Function4 : Trigonometry  Operator=cos
  Trigonometric Function5 : Trigonometry  Operator=cos
  Trigonometric Function6 : Trigonometry
  DQ : Outport
  wires:
  Mux1/1 -> DQ/1
  Product5/1 -> Sum6/3
  Constant2/1 -> Sum4/1
  Sum5/1 -> Trigonometric Function4/1
  Trigonometric Function4/1 -> Product4/2
  Trigonometric Function5/1 -> Product5/2
  Constant3/1 -> Sum5/1
  Sum6/1 -> Gain1/1
  Product3/1 -> Sum6/1
  Product4/1 -> Sum6/2
  Trigonometric Function3/1 -> Product3/2
  Gain1/1 -> Mux1/1
  ABC/1 -> Mux/1
  theta_d/1 -> Mux/2
  Demux/1 -> Product5/1
  Demux/2 -> Product4/1
  Demux/3 -> Product3/1
  Demux/4 -> Sum5/2, Trigonometric Function5/1, Sum4/2
  Mux/1 -> Demux/1, Demux1/1
  Sum4/1 -> Trigonometric Function3/1
  Product6/1 -> Sum3/3
  Constant1/1 -> Sum1/1
  Sum2/1 -> Trigonometric Function2/1
  Trigonometric Function2/1 -> Product2/2
  Trigonometric Function6/1 -> Product6/2
  Constant4/1 -> Sum2/1
  Sum3/1 -> Gain2/1
  Product1/1 -> Sum3/1
  Product2/1 -> Sum3/2
  Trigonometric Function1/1 -> Product1/2
  Gain2/1 -> Mux1/2
  Demux1/1 -> Product6/1
  Demux1/2 -> Product2/1
  Demux1/3 -> Product1/1
  Demux1/4 -> Sum1/2, Trigonometric Function6/1, Sum2/2
  Sum1/1 -> Trigonometric Function1/1

== system PTOSim_Lib_Updated/Generator/Direct Drive Linear Generator/Load ==
  Iabc : Inport
  Gain : Gain  Gain=-1
  Gain1 : Gain  Gain=ptosim.Rload
  Product : Product
  Sum of Elements : Sum  Inputs=+
  Vabc : Outport
  elecPower : Outport  Port=2
  wires:
  Gain/1 -> elecPower/1  "elecPower"
  Gain1/1 -> Product/1, Vabc/1
  Product/1 -> Sum of Elements/1
  Iabc/1 -> Gain1/1, Product/2
  Sum of Elements/1 -> Gain/1

== system PTOSim_Lib_Updated/Generator/Direct Drive Linear Generator/Losses ==
  vel : Inport
  Gain : Gain  Gain=ptosim.Bfric
  friceForce : Outport
  wires:
  vel/1 -> Gain/1
  Gain/1 -> friceForce/1

== system PTOSim_Lib_Updated/Generator/Direct Drive Linear Generator/Subsystem ==
  vsdq : Inport
  wd : Inport  Port=2
  Add : Sum  Inputs=+-+
  Add1 : Sum  Inputs=--+
  Demux2 : Demux  Outputs=2
      settings: DisplayOption=none
  Fcn : Fcn  Expr=( u(1) - ptosim.lambda_fd ) / ptosim.Ls
  Gain : Gain  Gain=1/ptosim.Ls
  Gain1 : Gain  Gain=pi/ptosim.tau_p*ptosim.lambda_fd
  Gain2 : Gain  Gain=ptosim.Rs
  Gain3 : Gain  Gain=ptosim.Rs
  Integrator : Integrator  InitialCondition=ptosim.lambda_sd_0
  Integrator1 : Integrator  InitialCondition=ptosim.lambda_sq_0
  Mux : Mux  Inputs=2
  Product : Product  RndMeth=Zero
  Product1 : Product  RndMeth=Zero
  Fem : Outport
  isdq : Outport  Port=2
  wires:
  Add/1 -> Integrator/1  "d_dt_lambda_sd"
  Integrator/1 -> Product1/2, Fcn/1  "lambda_sd"
  Fcn/1 -> Gain3/1, Mux/1  "isd"
  Product/1 -> Add/1
  Add1/1 -> Integrator1/1  "d_dt_lambda_sq"
  Integrator1/1 -> Gain/1, Product/2  "lambda_sq"
  wd/1 -> Product1/1, Product/1
  Gain/1 -> Gain2/1, Mux/2, Gain1/1  "isq"
  Product1/1 -> Add1/1
  Demux2/1 -> Add/3  "vsd"
  Demux2/2 -> Add1/3  "vsq"
  vsdq/1 -> Demux2/1  "vsdq"
  Gain3/1 -> Add/2  "isd_Rs"
  Gain2/1 -> Add1/2
  Mux/1 -> isdq/1  "isdq"
  Gain1/1 -> Fem/1

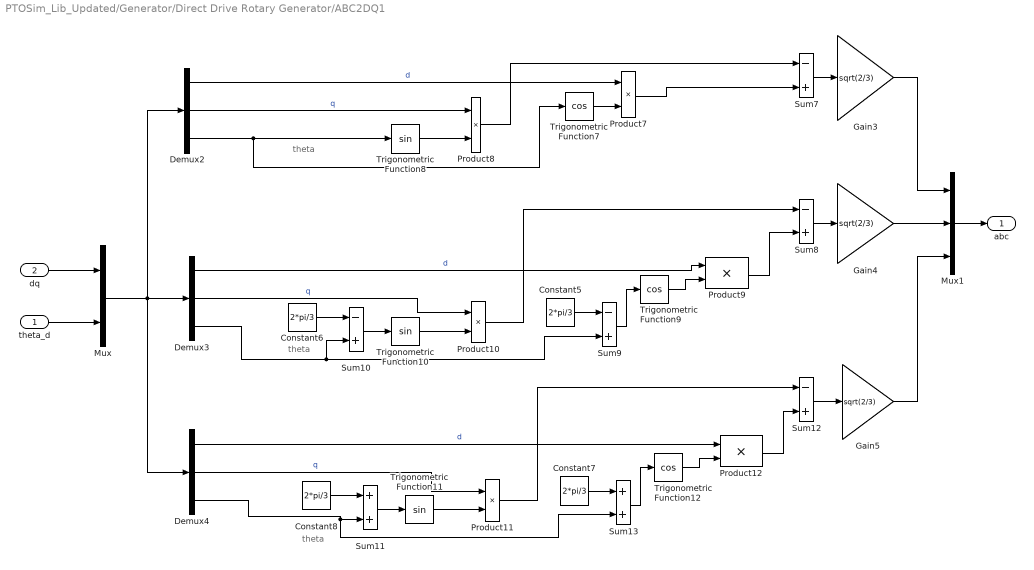
== system PTOSim_Lib_Updated/Generator/Direct Drive Rotary Generator/ABC2DQ1 ==
  note: theta
  note: theta
  note: theta
  theta_d : Inport
  dq : Inport  Port=2
  Constant{5..8} (4 alike) : Constant  Value=2*pi/3
  Demux2 : Demux  Outputs=3
      settings: DisplayOption=none
  Demux3 : Demux  Outputs=3
      settings: DisplayOption=none
  Demux4 : Demux  Outputs=3
      settings: DisplayOption=none
  Gain3 : Gain  Gain=sqrt(2/3)  SaturateOnIntegerOverflow=on  OutDataTypeStr=Inherit: Same as input  ParamDataTypeStr=Inherit: Same as input
  Gain4 : Gain  Gain=sqrt(2/3)  SaturateOnIntegerOverflow=on  OutDataTypeStr=Inherit: Same as input  ParamDataTypeStr=Inherit: Same as input
  Gain5 : Gain  Gain=sqrt(2/3)  SaturateOnIntegerOverflow=on  OutDataTypeStr=Inherit: Same as input  ParamDataTypeStr=Inherit: Same as input
  Mux : Mux  Inputs=2
  Mux1 : Mux  Inputs=3
  Product{7..12} (6 alike) : Product  InputSameDT=on  SaturateOnIntegerOverflow=on  OutDataTypeStr=Inherit: Same as first input
  Sum{7..10,12} (5 alike) : Sum  Inputs=-+  InputSameDT=on  SaturateOnIntegerOverflow=on  OutDataTypeStr=Inherit: Same as first input
  Sum11 : Sum  InputSameDT=on  SaturateOnIntegerOverflow=on  OutDataTypeStr=Inherit: Same as first input
  Sum13 : Sum  InputSameDT=on  SaturateOnIntegerOverflow=on  OutDataTypeStr=Inherit: Same as first input
  Trigonometric Function10 : Trigonometry
  Trigonometric Function11 : Trigonometry
  Trigonometric Function12 : Trigonometry  Operator=cos
  Trigonometric Function7 : Trigonometry  Operator=cos
  Trigonometric Function8 : Trigonometry
  Trigonometric Function9 : Trigonometry  Operator=cos
  abc : Outport
  wires:
  Mux1/1 -> abc/1
  dq/1 -> Mux/1
  theta_d/1 -> Mux/2
  Mux/1 -> Demux4/1, Demux2/1, Demux3/1
  Trigonometric Function7/1 -> Product7/2
  Demux2/1 -> Product7/1  "d"
  Product7/1 -> Sum7/2
  Product8/1 -> Sum7/1
  Demux2/3 -> Trigonometric Function8/1, Trigonometric Function7/1
  Demux2/2 -> Product8/1  "q"
  Trigonometric Function9/1 -> Product9/2
  Demux3/1 -> Product9/1  "d"
  Product9/1 -> Sum8/2
  Product10/1 -> Sum8/1
  Demux3/3 -> Sum10/2, Sum9/2
  Trigonometric Function10/1 -> Product10/2
  Demux3/2 -> Product10/1  "q"
  Sum9/1 -> Trigonometric Function9/1
  Constant5/1 -> Sum9/1
  Sum10/1 -> Trigonometric Function10/1
  Constant6/1 -> Sum10/1
  Trigonometric Function12/1 -> Product12/2
  Demux4/1 -> Product12/1  "d"
  Product12/1 -> Sum12/2
  Product11/1 -> Sum12/1
  Demux4/3 -> Sum13/2, Sum11/2
  Trigonometric Function11/1 -> Product11/2
  Demux4/2 -> Product11/1  "q"
  Sum13/1 -> Trigonometric Function12/1
  Constant7/1 -> Sum13/1
  Sum11/1 -> Trigonometric Function11/1
  Constant8/1 -> Sum11/1
  Sum7/1 -> Gain3/1
  Sum8/1 -> Gain4/1
  Sum12/1 -> Gain5/1
  Gain3/1 -> Mux1/1
  Gain4/1 -> Mux1/2
  Gain5/1 -> Mux1/3
  Trigonometric Function8/1 -> Product8/2

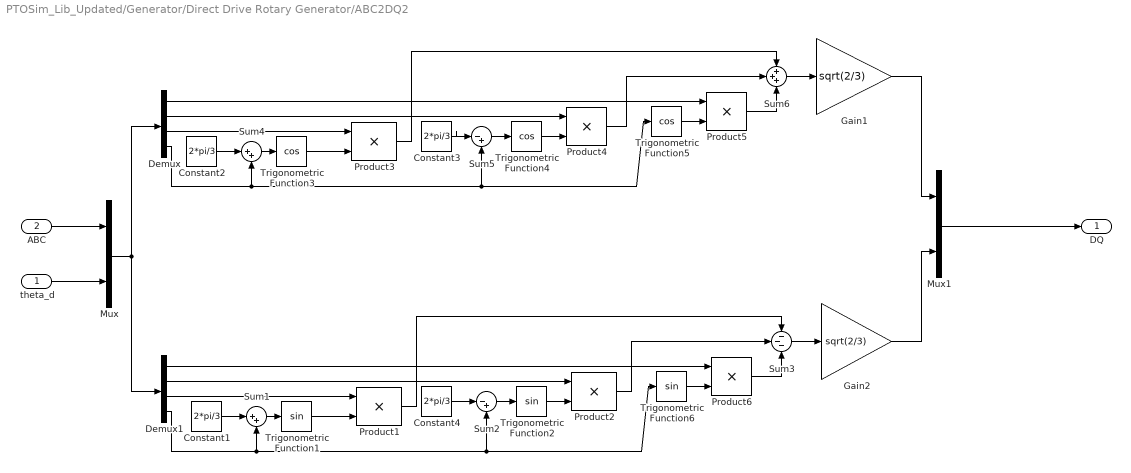
== system PTOSim_Lib_Updated/Generator/Direct Drive Rotary Generator/ABC2DQ2 ==
  theta_d : Inport
  ABC : Inport  Port=2
  Constant{1..4} (4 alike) : Constant  Value=2*pi/3
  Demux : Demux
      settings: DisplayOption=none
  Demux1 : Demux
      settings: DisplayOption=none
  Gain1 : Gain  Gain=sqrt(2/3)  SaturateOnIntegerOverflow=on  OutDataTypeStr=Inherit: Same as input  ParamDataTypeStr=Inherit: Same as input
  Gain2 : Gain  Gain=sqrt(2/3)  SaturateOnIntegerOverflow=on  OutDataTypeStr=Inherit: Same as input  ParamDataTypeStr=Inherit: Same as input
  Mux : Mux  Inputs=2
  Mux1 : Mux  Inputs=2
  Product{1..6} (6 alike) : Product  InputSameDT=on  SaturateOnIntegerOverflow=on  OutDataTypeStr=Inherit: Same as first input
  Sum1 : Sum  Inputs=|++  InputSameDT=on  SaturateOnIntegerOverflow=on  OutDataTypeStr=Inherit: Same as first input
  Sum2 : Sum  Inputs=|-+  InputSameDT=on  SaturateOnIntegerOverflow=on  OutDataTypeStr=Inherit: Same as first input
  Sum3 : Sum  Inputs=---  InputSameDT=on  SaturateOnIntegerOverflow=on  OutDataTypeStr=Inherit: Same as first input
  Sum4 : Sum  Inputs=|++  InputSameDT=on  SaturateOnIntegerOverflow=on  OutDataTypeStr=Inherit: Same as first input
  Sum5 : Sum  Inputs=|-+  InputSameDT=on  SaturateOnIntegerOverflow=on  OutDataTypeStr=Inherit: Same as first input
  Sum6 : Sum  Inputs=+++  InputSameDT=on  SaturateOnIntegerOverflow=on  OutDataTypeStr=Inherit: Same as first input
  Trigonometric Function1 : Trigonometry
  Trigonometric Function2 : Trigonometry
  Trigonometric Function3 : Trigonometry  Operator=cos
  Trigonometric Function4 : Trigonometry  Operator=cos
  Trigonometric Function5 : Trigonometry  Operator=cos
  Trigonometric Function6 : Trigonometry
  DQ : Outport
  wires:
  Mux1/1 -> DQ/1
  Product5/1 -> Sum6/3
  Constant2/1 -> Sum4/1
  Sum5/1 -> Trigonometric Function4/1
  Trigonometric Function4/1 -> Product4/2
  Trigonometric Function5/1 -> Product5/2
  Constant3/1 -> Sum5/1
  Sum6/1 -> Gain1/1
  Product3/1 -> Sum6/1
  Product4/1 -> Sum6/2
  Trigonometric Function3/1 -> Product3/2
  Gain1/1 -> Mux1/1
  ABC/1 -> Mux/1
  theta_d/1 -> Mux/2
  Demux/1 -> Product5/1
  Demux/2 -> Product4/1
  Demux/3 -> Product3/1
  Demux/4 -> Sum5/2, Trigonometric Function5/1, Sum4/2
  Mux/1 -> Demux/1, Demux1/1
  Sum4/1 -> Trigonometric Function3/1
  Product6/1 -> Sum3/3
  Constant1/1 -> Sum1/1
  Sum2/1 -> Trigonometric Function2/1
  Trigonometric Function2/1 -> Product2/2
  Trigonometric Function6/1 -> Product6/2
  Constant4/1 -> Sum2/1
  Sum3/1 -> Gain2/1
  Product1/1 -> Sum3/1
  Product2/1 -> Sum3/2
  Trigonometric Function1/1 -> Product1/2
  Gain2/1 -> Mux1/2
  Demux1/1 -> Product6/1
  Demux1/2 -> Product2/1
  Demux1/3 -> Product1/1
  Demux1/4 -> Sum1/2, Trigonometric Function6/1, Sum2/2
  Sum1/1 -> Trigonometric Function1/1

== system PTOSim_Lib_Updated/Generator/Direct Drive Rotary Generator/Load ==
  Iabc : Inport
  Gain : Gain  Gain=-1
  Gain1 : Gain  Gain=ptosim.Rload
  Product : Product
  Sum of Elements : Sum  Inputs=+
  Vabc : Outport
  elecPower : Outport  Port=2
  wires:
  Gain/1 -> elecPower/1  "elecPower"
  Gain1/1 -> Product/1, Vabc/1
  Product/1 -> Sum of Elements/1
  Iabc/1 -> Gain1/1, Product/2
  Sum of Elements/1 -> Gain/1

== system PTOSim_Lib_Updated/Generator/Direct Drive Rotary Generator/Losses ==
  vel : Inport
  Gain : Gain  Gain=ptosim.Bfric
  fricTorque : Outport
  wires:
  vel/1 -> Gain/1
  Gain/1 -> fricTorque/1
